simulink model "Spike_Generator"  (R2019b)
settings: Solver=VariableStepAuto  StartTime=0.0  StopTime=testtime  RelTol=1e-3
InitFcn:
  | Spike_Generator_Test_Parameters
StopFcn:
  | Verify_Spike_Generator
values from neighbouring files (symbols this model uses):
  Fs = 48e3    (= 48000)    [Spike_Generator_Test_Parameters.m]
  nSites = 4    [Spike_Generator_Test_Parameters.m]
  tabs = 0.6e-3    (= 0.0006)    [Spike_Generator_Test_Parameters.m]
  trel = 0.6e-3    (= 0.0006)    [Spike_Generator_Test_Parameters.m]
libraries: dspsrcs4 x4
(part 3 of 3)

== stateflow chart Spike_Generator/Spike Generator Doubles/Stateflow Logic Chart ==
  settings: updateMethod=DISCRETE  sampleTime=tdres  executeAtInitialization=1
  note: 1st Synaptic Site State
      |
      | - Updates according to whether the synaptic site is sensing input or is going through the redocking period.
  note: 2nd Synaptic Site State
      |
      | - Updates according to whether the synaptic site is sensing input or is going through the redocking period.
  note: 3rd Synaptic Site State
      |
      | - Updates according to whether the synaptic site is sensing input or is going through the redocking period.
  note: 4th Synaptic Site State
      |
      | - Updates according to whether the synaptic site is sensing input or is going through the redocking period.
  note: Redocking Decay State
      |
      | - Updates according to whether the redocking period should be decayed or a redocking event has occured during the time step
  note: Synaptic State
      |
      | - Updates according to whether the synapse is ready to fire or is going through the refractory period.
  state SynapticSite1 [parallel]
    settings: executionOrder=2
    note: Synaptic Site Sensing Input
    note: Synaptic Site In Redocking Period
    note: Default Transition
    state SenseInput
      entry:
      redockStatus1 = 0;
      Xsum1 = Xsum1 + synoutdouble/4;
      releaseStatus1 = checkRelease(Xsum1, unitRateInterval1);
      during:
      Xsum1 = Xsum1 + synoutdouble/4;
      releaseStatus1 = checkRelease(Xsum1, unitRateInterval1);
      exit:
      oneSiteRedock1 = getNewRedock(current_redocking_period, randNumsdouble);
      Xsum1= 0;
      unitRateInterval1 = getNewUnitRateInterval(randNumsdouble);
    state RedockPeriod
      entry:
      elapsed_time1 = 0;
      redockStatus1 = checkRedock(elapsed_time1, oneSiteRedock1);
      elapsed_time1  = elapsed_time1 + tdres;
      releaseStatus1 = 0;
      during:
      redockStatus1 = checkRedock(elapsed_time1, oneSiteRedock1);
      elapsed_time1 = elapsed_time1 + tdres;
      exit:
      elapsed_time1 = 0;
      current_redocking_period = previous_redocking_period + t_rd_jump;
      previous_redocking_period = current_redocking_period;
    (default) -> SynapticSite1.RedockPeriod
    SynapticSite1.SenseInput -> SynapticSite1.RedockPeriod : [releaseStatus1 == 1]
    SynapticSite1.RedockPeriod -> SynapticSite1.SenseInput : [redockStatus1 == 1]
  state SynapticSite2 [parallel]
    settings: executionOrder=3
    note: Synaptic Site Sensing Input
    note: Synaptic Site In Redocking Period
    note: Default Transition
    state SenseInput
      entry:
      redockStatus2 = 0;
      Xsum2 = Xsum2 + synoutdouble/4;
      releaseStatus2 = checkRelease(Xsum2, unitRateInterval2);
      during:
      Xsum2 = Xsum2 + synoutdouble/4;
      releaseStatus2 = checkRelease(Xsum2, unitRateInterval2);
      exit:
      oneSiteRedock2 = getNewRedock(current_redocking_period, randNumsdouble);
      Xsum2= 0;
      unitRateInterval2 = getNewUnitRateInterval(randNumsdouble);
    state RedockPeriod
      entry:
      elapsed_time2 = 0;
      redockStatus2 = checkRedock(elapsed_time2, oneSiteRedock2);
      elapsed_time2  = elapsed_time2 + tdres;
      releaseStatus2 = 0;
      during:
      redockStatus2 = checkRedock(elapsed_time2, oneSiteRedock2);
      elapsed_time2 = elapsed_time2 + tdres;
      exit:
      elapsed_time2 = 0;
      current_redocking_period = previous_redocking_period + t_rd_jump;
      previous_redocking_period = current_redocking_period;
    (default) -> SynapticSite2.RedockPeriod
    SynapticSite2.SenseInput -> SynapticSite2.RedockPeriod : [releaseStatus2 == 1]
    SynapticSite2.RedockPeriod -> SynapticSite2.SenseInput : [redockStatus2 == 1]
  state SynapticSite3 [parallel]
    settings: executionOrder=4
    note: Synaptic Site Sensing Input
    note: Synaptic Site In Redocking Period
    note: Default Transition
    state SenseInput
      entry:
      redockStatus3 = 0;
      Xsum3 = Xsum3 + synoutdouble/4;
      releaseStatus3 = checkRelease(Xsum3, unitRateInterval3);
      during:
      Xsum3 = Xsum3 + synoutdouble/4;
      releaseStatus3 = checkRelease(Xsum3, unitRateInterval3);
      exit:
      oneSiteRedock3 = getNewRedock(current_redocking_period, randNumsdouble);
      Xsum3= 0;
      unitRateInterval3 = getNewUnitRateInterval(randNumsdouble);
    state RedockPeriod
      entry:
      elapsed_time3 = 0;
      redockStatus3 = checkRedock(elapsed_time3, oneSiteRedock3);
      elapsed_time3  = elapsed_time3 + tdres;
      releaseStatus3 = 0;
      during:
      redockStatus3 = checkRedock(elapsed_time3, oneSiteRedock3);
      elapsed_time3 = elapsed_time3 + tdres;
      exit:
      elapsed_time3 = 0;
      current_redocking_period = previous_redocking_period + t_rd_jump;
      previous_redocking_period = current_redocking_period;
    (default) -> SynapticSite3.RedockPeriod
    SynapticSite3.SenseInput -> SynapticSite3.RedockPeriod : [releaseStatus3 == 1]
    SynapticSite3.RedockPeriod -> SynapticSite3.SenseInput : [redockStatus3 == 1]
  state SynapticSite4 [parallel]
    settings: executionOrder=5
    note: Synaptic Site Sensing Input
    note: Synaptic Site In Redocking Period
    note: Default Transition
    state SenseInput
      entry:
      redockStatus4 = 0;
      Xsum4 = Xsum4 + synoutdouble/4;
      releaseStatus4 = checkRelease(Xsum4, unitRateInterval4);
      during:
      Xsum4 = Xsum4 + synoutdouble/4;
      releaseStatus4 = checkRelease(Xsum4, unitRateInterval4);
      exit:
      oneSiteRedock4 = getNewRedock(current_redocking_period, randNumsdouble);
      Xsum4= 0;
      unitRateInterval4 = getNewUnitRateInterval(randNumsdouble);
    state RedockPeriod
      entry:
      elapsed_time4 = 0;
      redockStatus4 = checkRedock(elapsed_time4, oneSiteRedock4);
      elapsed_time4  = elapsed_time4 + tdres;
      releaseStatus4 = 0;
      during:
      redockStatus4 = checkRedock(elapsed_time4, oneSiteRedock4);
      elapsed_time4 = elapsed_time4 + tdres;
      exit:
      elapsed_time4 = 0;
      current_redocking_period = previous_redocking_period + t_rd_jump;
      previous_redocking_period = current_redocking_period;
    (default) -> SynapticSite4.RedockPeriod
    SynapticSite4.SenseInput -> SynapticSite4.RedockPeriod : [releaseStatus4 == 1]
    SynapticSite4.RedockPeriod -> SynapticSite4.SenseInput : [redockStatus4 == 1]
  state RedockingDecay [parallel]
    settings: executionOrder=6
    note: Decay Redocking Period
    note: Don't Decay Redocking Period
    note: Default Transition
    state DecayRedockingPeriod
      entry:
      current_redocking_period = decayRedock(previous_redocking_period, tdres, tau, t_rd_rest);
      previous_redocking_period = current_redocking_period;
      trd_vector = current_redocking_period;
      during:
      current_redocking_period = decayRedock(previous_redocking_period, tdres, tau, t_rd_rest);
      previous_redocking_period = current_redocking_period;
      trd_vector = current_redocking_period;
    state NoDecay
      entry:
      trd_vector = current_redocking_period;
      during:
      trd_vector = current_redocking_period;
    (default) -> DecayRedockingPeriod
    DecayRedockingPeriod -> NoDecay : [redockStatus1 == 1 || redockStatus2 == 1 || redockStatus3 == 1 || redockStatus4 == 1]
    NoDecay -> DecayRedockingPeriod : [redockStatus1 == 0 && redockStatus2 == 0 && redockStatus3 == 0 && redockStatus4 == 0]
  state Synapse [parallel]
    settings: executionOrder=1
    note: Synapse Ready to Fire
    note: Synapse in Refractory Period
    note: Default Transition
    state RefractoryPeriod
      entry:
      refractoryStatus = checkRefractory(refractory_time, Tref);
      refractory_time = refractory_time + tdres;
      during:
      sptime = 0;
      refractoryStatus = checkRefractory(refractory_time, Tref);
      refractory_time = refractory_time + tdres;
      exit:
      refractory_time = 0;
      sptime = 0;
    state SynapseReady
      during:
      sptime = 0;
      exit:
      sptime = 1;
      spCount = spCount + 1;
      Tref = getTref(synoutdouble, randNumsdouble, trel, tabs);
    (default) -> SynapseReady
    SynapseReady -> RefractoryPeriod : [releaseStatus1 == 1 || releaseStatus2 ==1 || releaseStatus3 == 1 || releaseStatus4 ==1]
    RefractoryPeriod -> SynapseReady : [refractoryStatus == 0]
  note: Release Status Graphical Function
      |
      | Input : Sensing Input Sum (Xsum) & Release Threshold (unitRateInterval)
      |
      | Output : Release Status Condition (releaseStatus)
      |
      | - Checks if a Release Event Occurs for the Synaptic Site (1) or not (0)
  state releaseStatuscond = checkRelease(Xsumval, unitRateIntervalval) [function]
    (default) -> (junction 138) : % Check to see if a release event occurs.
    (junction 138) -> (junction 139) [order 1] : [Xsumval >= unitRateIntervalval]
    (junction 138) -> (junction 140) [order 2] : {releaseStatuscond = 0;}
    (junction 139) -> (junction 141) : {releaseStatuscond = 1;}
    (junction 141) -> (junction 140)
    (junction 140) -> (junction 142)
  state redockStatuscond = checkRedock(elapsed_timeval, oneSiteRedockval) [function]
    (default) -> (junction 153) : % Check to see if a redocking event occurs.
    (junction 153) -> (junction 154) [order 1] : [elapsed_timeval >= oneSiteRedockval]
    (junction 153) -> (junction 155) [order 2] : {redockStatuscond = 0;}
    (junction 154) -> (junction 156) : {redockStatuscond = 1;}
    (junction 156) -> (junction 155)
    (junction 155) -> (junction 157)
  note: Redock Status Graphical Function
      |
      | Input : Elapsed Time during Redocking Event (elapsed_time) & Site Specific Redocking Period (oneSiteRedock)
      |
      | Output : Redock Status Condition (redockStatus)
      |
      | - Checks if a Redocking Event Occurs for the Synaptic Site (1) or not (0)
  state refractoryStatuscond = checkRefractory(refractory_timeval, Trefval) [function]
    (default) -> (junction 272) : % Check to see if the synapse is in the refractory period.
    (junction 272) -> (junction 273) [order 1] : [refractory_timeval >= Trefval]
    (junction 272) -> (junction 274) [order 2] : {refractoryStatuscond = 1;}
    (junction 273) -> (junction 275) : {refractoryStatuscond = 0;}
    (junction 275) -> (junction 274)
    (junction 274) -> (junction 276)
  note: Refractory Status Graphical Function
      |
      | Input : Elapsed Time during Refractory Period (refractory_time) & Refractory Period (Tref)
      |
      | Output : Refractory Status Condition (refractoryStatus)
      |
      | - Checks if the Synapse is in the Refractory Period (1) or not (0)
  note: Get New Unit Rate Interval MATLAB Function
      |
      | Input : Uniformly Distributed Random Number between 0 and 1 (randNums)
      |
      | Output : New Release Threshold Value (unitRateInterval)
      |
      | - Calculates the New Release Threshold Value for the Synaptic Site after a Release Event
  note: Get New Site Specific Redocking Period MATLAB Function
      |
      | Input : Current Redocking Period (current_redocking_period) & Uniformly Distributed Random Number between 0 and 1 (randNums)
      |
      | Output : New Redocking Period for Specific Synaptic Site (oneSiteRedock)
      |
      | - Calculates the New Redocking Period for Specific Synaptic Site
  note: Decay Redocking Period MATLAB Function
      |
      | Input : Previous Redocking Period (previous_redocking_period), Sample Time (tdres),
      | Decay Time Constant (tau), & Resting Redocking Time (t_rd_rest)
      |
      | Output : Current Redocking Period (current_redocking_period)
      |
      | - Decays the Redocking Period for the Next TIme Step
  note: Get New Refractory Period MATLAB Function
      |
      | Input : Synapse Output (synout), Uniformly Distributed Random Number between 0 and 1 (randNums),
      | Relative Refractory Time (trel), & Absolute Refractory Time (tabs)
      |
      | Output : New Refractory Period for the Synapse (Tref)
      |
      | - Calculates the New Refractory Period for the Synapse
  data: Xsumval function_input; releaseStatuscond function_output; unitRateIntervalval function_input; elapsed_timeval function_input; redockStatuscond function_output; oneSiteRedockval function_input; refractory_timeval function_input; refractoryStatuscond function_output; Trefval function_input; randNumsval function_input; unitRateIntervalval function_output; current_redocking_periodval function_input; randNumsval function_input; oneSiteRedockval function_output; previous_redocking_periodval function_input; current_redocking_periodval function_output; tdresval function_input; tauval function_input; t_rd_restval function_input; synoutval function_input; Trefval function_output; randNumsval function_input; trelval function_input; tabsval function_input; tdres parameter; synoutdouble input; refractoryStatus local; randNumsdouble input; sptime output; spCount output; current_redocking_period output; trd_vector output; t_rd_jump parameter; releaseStatus1 local; redockStatus1 local; releaseStatus4 local; redockStatus4 local; releaseStatus2 local; redockStatus2 local; releaseStatus3 local; redockStatus3 local; t_rd_rest parameter; tau parameter; trel parameter; tabs parameter; unitRateInterval4 local; unitRateInterval3 local; unitRateInterval2 local; unitRateInterval1 local; oneSiteRedock4 local; oneSiteRedock3 local; oneSiteRedock2 local; oneSiteRedock1 local; elapsed_time4 local; elapsed_time3 local; elapsed_time2 local; elapsed_time1 local; Xsum4 local; Xsum3 local; Xsum2 local; Xsum1 local; Tref local; previous_redocking_period local; refractory_time local
  function unitRateIntervalval = getNewUnitRateInterval(randNumsval):
    | function unitRateIntervalval = getNewUnitRateInterval(randNumsval)
    |     unitRateIntervalval = -log(randNumsval)/tdres;
    | end
  function oneSiteRedockval = getNewRedock(current_redocking_periodval, randNumsval):
    | function oneSiteRedockval = getNewRedock(current_redocking_periodval, randNumsval)
    |     oneSiteRedockval = -current_redocking_periodval * log(randNumsval);
    | end
  function current_redocking_periodval = decayRedock(previous_redocking_periodval,tdresval,tauval,t_rd_restval):
    | function current_redocking_periodval = decayRedock(previous_redocking_periodval,tdresval,tauval,t_rd_restval)
    |     current_redocking_periodval = previous_redocking_periodval - (tdresval/tauval)*(previous_redocking_periodval - t_rd_restval);
    | end
  function Trefval = getTref(synoutval, randNumsval, trelval, tabsval):
    | function Trefval = getTref(synoutval, randNumsval, trelval, tabsval)
    |     trel_k = min(trelval*100/synoutval,trelval);
    |     Trefval = tabsval - trel_k*log(randNumsval); 
    | end
